simulink model "ParameterEstimation"  (R2025b)
settings: Solver=ode45  StartTime=0.0  StopTime=1  RelTol=1e-3  EnableMultiTasking=on
InitFcn:
  | ts = prepareLogForParameterEstimation("../LOGS/log0168.csv")
settings Model: ModifiedByFormat=The MathWorks Inc.  Creator=The MathWorks, Inc.  LastModifiedBy=The MathWorks Inc.
settings SolverCC: AlgebraicLoopSolver=TrustRegion
settings DataIOCC: LimitDataPoints=on  SaveFormat=Array  SaveOutput=off  SaveTime=off  ReturnWorkspaceOutputs=off
settings OptimizationCC: ExpressionDepthLimit=2147483647.0  LifeSpan=1
settings DebuggingCC: UnderspecifiedInitializationDetection=Classic  MergeDetectMultiDrivingBlocksExec=none  SolverPrmCheckMsg=warning  FcnCallInpInsideContextMsg=warning  UnconnectedInputMsg=warning  UnconnectedOutputMsg=warning  UnconnectedLineMsg=warning  StateNameClashWarn=warning  SFUnexpectedBacktrackingDiag=warning  SFNoUnconditionalDefaultTransitionDiag=warning  SFExecutionAtInitializationDiag=none  ArithmeticOperatorsInVariantConditions=warning
settings HardwareCC: ProdBitPerPointer=32.0  ProdBitPerSizeT=32.0  ProdBitPerPtrDiffT=32.0  ProdLargestAtomicFloat=None  ProdIntDivRoundTo=Undefined  ProdEndianess=Unspecified  ProdWordSize=32.0  ProdHWDeviceType=32-bit Generic
settings ModelReferenceCC: PropagateSignalLabelsOutOfModel=off
settings SFSimCC: SimUseLocalCustomCode=off  CustomCodeUndefinedFunction=UseInterfaceOnly
settings RTWCC: RTWUseLocalCustomCode=off  GPUComputeCapability=3.5
settings CodeAppCC: StateflowObjectComments=on
settings GRTTargetCC: TargetLangStandard=C89/C90 (ANSI)  CombineOutputUpdateFcns=off  GRTInterface=on
settings ConfigComp: CovMetricSettings=dw  CovSaveCumulativeToWorkspaceVar=on  CovSaveSingleToWorkspaceVar=on  CovExternalEMLEnable=off  CovSFcnEnable=off

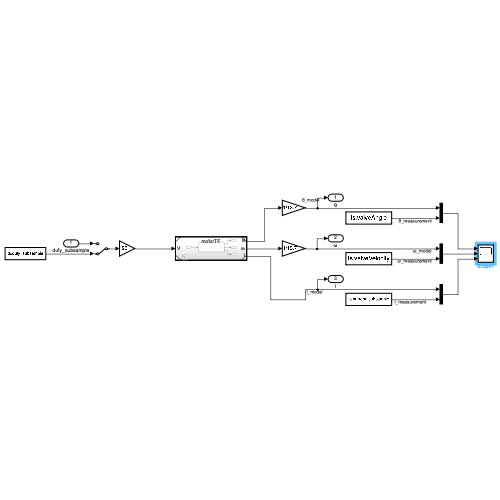
[thumbnail: Simulink's stored preview of the top-level diagram]
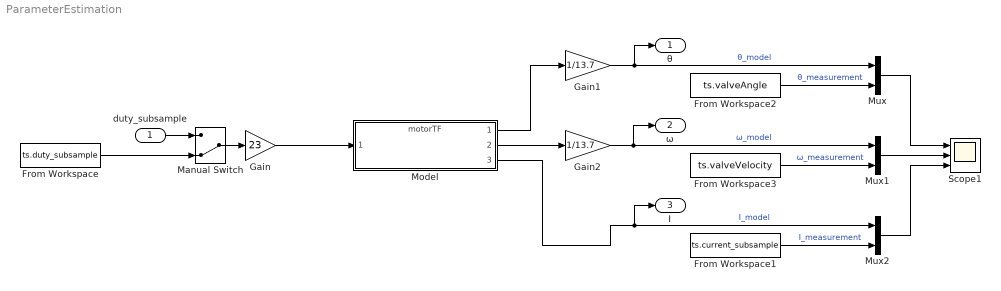
== system ParameterEstimation ==
  duty_subsample : Inport
  From Workspace : FromWorkspace  VariableName=ts.duty_subsample
  From Workspace1 : FromWorkspace  VariableName=ts.current_subsample
  From Workspace2 : FromWorkspace  VariableName=ts.valveAngle
  From Workspace3 : FromWorkspace  VariableName=ts.valveVelocity
  Gain : Gain  Gain=23
  Gain1 : Gain  Gain=1/13.7
  Gain2 : Gain  Gain=1/13.7
  Manual Switch : ManualSwitch  CurrentSetting=0
  Model : ModelReference  ModelNameDialog=motorTF.slx  SimulationMode=Normal  ModelReferenceVersion=1.3
  Mux : Mux  Inputs=2
  Mux1 : Mux  Inputs=2
  Mux2 : Mux  Inputs=2
  Scope1 : Scope  NumInputPorts=3
      settings: TimeSpan=1  ActiveDisplayYMinimum=-228.23083119215482  ActiveDisplayYMaximum=2053.8358514130769
  θ : Outport  Unit=deg
  ω : Outport  Port=2  Unit=deg/s
  I : Outport  Port=3  Unit=A
  wires:
  Gain/1 -> Model/1
  Model/3 -> I/1, Mux2/1  "I_model"
  duty_subsample/1 -> Manual Switch/1
  From Workspace/1 -> Manual Switch/2
  Manual Switch/1 -> Gain/1
  Model/2 -> Gain2/1
  Model/1 -> Gain1/1
  From Workspace1/1 -> Mux2/2  "I_measurement"
  From Workspace2/1 -> Mux/2  "θ_measurement"
  From Workspace3/1 -> Mux1/2  "ω_measurement"
  Gain1/1 -> θ/1, Mux/1  "θ_model"
  Gain2/1 -> ω/1, Mux1/1  "ω_model"
  Mux1/1 -> Scope1/2
  Mux/1 -> Scope1/1
  Mux2/1 -> Scope1/3
